simulink model "PN_generator_Tx"  (R2020a)
settings: Solver=FixedStepAuto  StartTime=0.0  StopTime=60  RelTol=1e-3  EnableMultiTasking=on
undefined symbols (not defined in the file): Fs, ip, usb
libraries: commfilt2 x6, commdigbbndpm3 x3, plutoradiolib x2, commseqgen3 x1, commutil2 x1
settings Model: DataTypeOverride=Off  Creator=juanj  LastModifiedBy=juanj
settings SolverCC: PositivePriorityOrder=on
settings OptimizationCC: BlockReduction=off  ConditionallyExecuteInputs=off  EnhancedBackFolding=on  PassReuseOutputArgsAs=Individual arguments  ZeroExternalMemoryAtStartup=off  ZeroInternalMemoryAtStartup=off  MaxStackSize=64  OptimizeBlockOrder=speed  DifferentSizesBufferReuse=on  OptimizationCustomize=off  EfficientTunableParamExpr=on
settings DebuggingCC: SignalRangeChecking=warning  AlgebraicLoopMsg=error  SingleTaskRateTransMsg=error  ParameterTunabilityLossMsg=error  SFUnexpectedBacktrackingDiag=warning  SFNoUnconditionalDefaultTransitionDiag=warning  UnderSpecifiedDimensionMsg=warning
settings HardwareCC: ProdBitPerPointer=32  ProdBitPerSizeT=32  ProdBitPerPtrDiffT=32  ProdLargestAtomicInteger=Long  ProdLargestAtomicFloat=Double  ProdWordSize=32  ProdLongLongMode=on  ProdHWDeviceType=ARM Compatible->ARM Cortex  TargetBitPerPointer=64  TargetBitPerSizeT=64  TargetBitPerPtrDiffT=64  TargetLongLongMode=on  TargetIntDivRoundTo=Zero  TargetEndianess=LittleEndian  TargetWordSize=64  TargetHWDeviceType=Custom Processor->MATLAB Host Computer  ProdEqTarget=off
settings SFSimCC: MATLABDynamicMemAlloc=off
settings RTWCC: SystemTargetFile=ert.tlc  HardwareBoard=ZedBoard  TemplateMakefile=ert_default_tmf  GenerateReport=on  Toolchain=Linaro AArch32 Linux v6.3.1  BuildConfiguration=Debug  LaunchReport=on
settings CodeAppCC: ForceParamTrailComments=on  IgnoreCustomStorageClasses=off  OperatorAnnotations=on  SimulinkDataObjDesc=on  SFDataObjDesc=on  InsertBlockDesc=on  EnableCustomComments=on

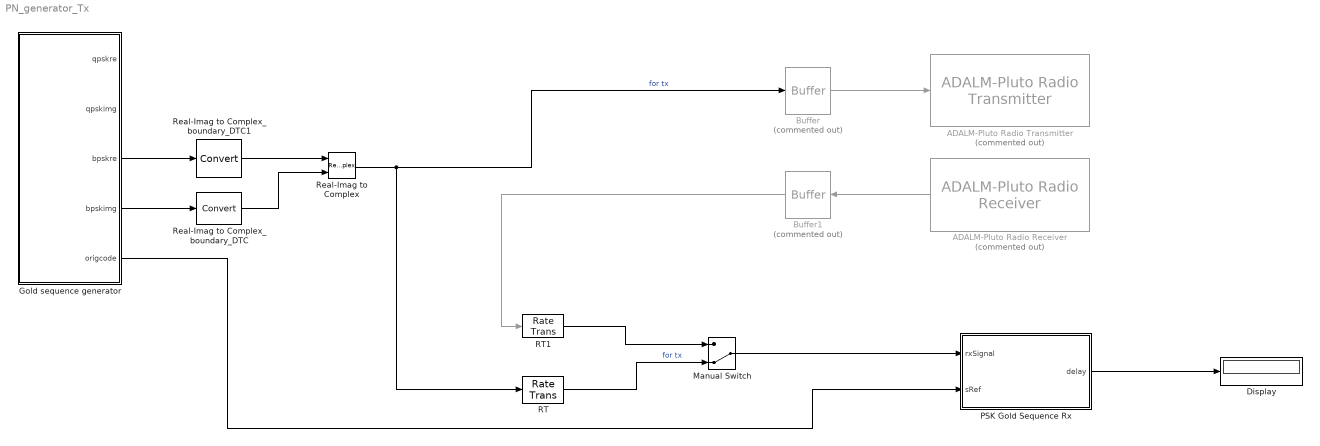
== system PN_generator_Tx ==
  ADALM-Pluto Radio Receiver : plutoradiolib/ADALM-Pluto Radio Receiver  Commented=on  RadioID=usb:0  uri=ip:10.0.0.200  CenterFrequencySource=Dialog  CenterFrequency=900e6  GainSource=AGC Slow Attack  GainSourceBlock=AGC Slow Attack  Gain=10  ChannelMapping=1  BasebandSampleRate=0.5e6  OutputDataType=double  SamplesPerFrame=11216  OverflowOutputPort=off  EnableBurstMode=off  NumFramesInBurst=1  ShowAdvancedProperties=off  UseCustomFilter=off  filtPathRates=[737280000 11520000 3840000 1920000 960000 240000]  filtCoefficients=[-192 82 85 -215 228 -102 -110 290 -318 145 160 -426 471 -215 -238 633 -697 318 349 -923 1009 -457 -498 1309 -1423 640 693 -1812 1959 -876 -945 2458 -2647 1180 1268 -3290 3534 -1572 -1688 4375 -4698 2091 2247 -5836 6284 -2807 -3031 7918 -8588 3870 4225 -11182 12324 -5662 -6330 17255 -19735 9507 11312 -33568 43355 -25227 -42139 305542 305542 -42139 -25227 43355 -33568 11312 9507 -19735 17255 -6330 -5662 12324 -11182 4225 3870 -8588 7918 -3031 -2807 6284 -5836 2247 2091 -4698 4375 -1688 -1572 3534 -3290 1268 1180 -2647 2458 -945 -876 1959 -1812 693 640 -1423 1309 -498 -457 1009 -923 349 318 -697 633 -238 -215 471 -426 160 145 -318 290 -110 -102 228 -215 85 82 -192]  filtCoefficientSize=128  filtDecimInterpFactor=4  filtGain=-12  filtRFBandwidth=18000000  filterConfigStruct=struct()  EnableQuadratureCorrection=on  EnableRFDCCorrection=on  EnableBasebandDCCorrection=on  FrequencyCorrection=0  OverrideSampleTime=off  SampleTime=0.02  DataTimeout=Inf  ENSMPinControlMode=None  BISTLoopbackMode=Disabled  BISTToneInject=Disabled  BISTSignalGen=PRBS  BISTToneFreq=Fs/32  BISTToneLevel=0
      settings: SourceProductBaseCode=PLUTO
  ADALM-Pluto Radio Transmitter : plutoradiolib/ADALM-Pluto Radio Transmitter  Commented=on  RadioID=usb:0  uri=ip:10.0.0.200  CenterFrequencySource=Dialog  CenterFrequency=900e6  GainSource=Dialog  Gain=0  ChannelMapping=1  BasebandSampleRate=0.5e6  UnderflowOutputPort=off  ShowAdvancedProperties=off  UseCustomFilter=off  filtPathRates=[737280000 11520000 3840000 1920000 960000 240000]  filtCoefficients=[-192 82 85 -215 228 -102 -110 290 -318 145 160 -426 471 -215 -238 633 -697 318 349 -923 1009 -457 -498 1309 -1423 640 693 -1812 1959 -876 -945 2458 -2647 1180 1268 -3290 3534 -1572 -1688 4375 -4698 2091 2247 -5836 6284 -2807 -3031 7918 -8588 3870 4225 -11182 12324 -5662 -6330 17255 -19735 9507 11312 -33568 43355 -25227 -42139 305542 305542 -42139 -25227 43355 -33568 11312 9507 -19735 17255 -6330 -5662 12324 -11182 4225 3870 -8588 7918 -3031 -2807 6284 -5836 2247 2091 -4698 4375 -1688 -1572 3534 -3290 1268 1180 -2647 2458 -945 -876 1959 -1812 693 640 -1423 1309 -498 -457 1009 -923 349 318 -697 633 -238 -215 471 -426 160 145 -318 290 -110 -102 228 -215 85 82 -192]  filtCoefficientSize=128  filtDecimInterpFactor=4  filtGain=-12  filtRFBandwidth=18000000  filterConfigStruct=struct()  DataSourceSelect=Input Port  DDSTone1Freq=5e3  DDSTone2Freq=10e3  DDSTone1Scale=0.5  DDSTone2Scale=0.25  DataTimeout=Inf  FrequencyCorrection=0  ENSMPinControlMode=None  BISTLoopbackMode=Disabled  BISTToneInject=Disabled  BISTSignalGen=PRBS  BISTToneFreq=Fs/32  BISTToneLevel=0
      settings: SourceProductBaseCode=PLUTO
  Buffer : Buffer  Commented=on  N=11216  OutputFrames=off
  Buffer1 : Buffer  Commented=on  N=1  OutputFrames=off
  Display : Display
  Gold sequence generator : Subsystem  TreatAsAtomicUnit=on
  Manual Switch : ManualSwitch  CurrentSetting=0
  PSK Gold Sequence Rx : Subsystem
  RT : RateTransition
  RT1 : RateTransition
  Real-Imag to Complex : RealImagToComplex
  Real-Imag to Complex_boundary_DTC : DataTypeConversion  SaturateOnIntegerOverflow=on  RndMeth=Zero
  Real-Imag to Complex_boundary_DTC1 : DataTypeConversion  SaturateOnIntegerOverflow=on  RndMeth=Zero
  wires:
  Real-Imag to Complex/1 -> RT/1, Buffer/1  "for tx"
  Buffer/1 -> ADALM-Pluto Radio Transmitter/1
  Gold sequence generator/4(bpskimg) -> Real-Imag to Complex_boundary_DTC/1
  Real-Imag to Complex_boundary_DTC/1 -> Real-Imag to Complex/2
  Gold sequence generator/3(bpskre) -> Real-Imag to Complex_boundary_DTC1/1
  Real-Imag to Complex_boundary_DTC1/1 -> Real-Imag to Complex/1
  Gold sequence generator/5(origcode) -> PSK Gold Sequence Rx/2(sRef)
  RT/1 -> Manual Switch/2  "for tx"
  ADALM-Pluto Radio Receiver/1 -> Buffer1/1
  Buffer1/1 -> RT1/1
  RT1/1 -> Manual Switch/1
  PSK Gold Sequence Rx/1(delay) -> Display/1
  Manual Switch/1 -> PSK Gold Sequence Rx/1(rxSignal)

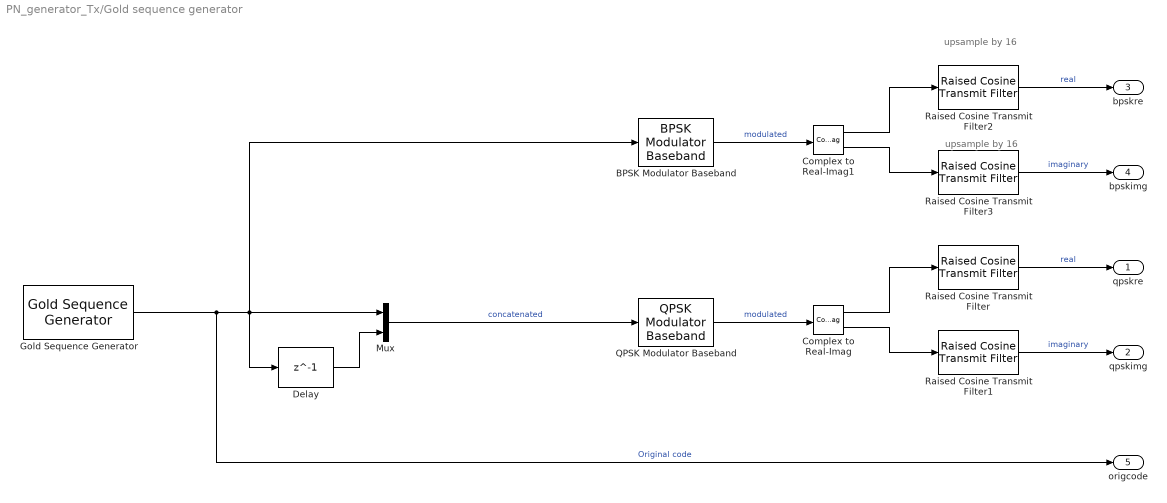
== system PN_generator_Tx/Gold sequence generator ==
  note: upsample by 16
  note: upsample by 16
  BPSK Modulator Baseband : commdigbbndpm3/BPSK Modulator Baseband  Ph=0  outDtype=Fixed-point  outWordLen=16  outUDDataType=sfix(16)  outFracLenMode=Best precision  outFracLen=15  outDataTypeStr=fixdt(1,16)  outLastDataTypeStr=fixdt(1,16)
  Complex to Real-Imag : ComplexToRealImag
  Complex to Real-Imag1 : ComplexToRealImag
  Delay : Delay  DelayLength=1  InitialCondition=0  UseCircularBuffer=on
  Gold Sequence Generator : commseqgen3/Gold Sequence Generator  genPoly1='z^6 + z + 1'  iniState1=[0 1 0 1 0 1]  genPoly2='z^6 + z^5 + z^2 + z + 1'  iniState2=[0 0 0 0 0 1]  index=0  shift=0  outVarSiz=off  maxOutSizeMode=Dialog parameter  maxOutSize=[10 1]  Ts=1/100  sampPerFrame=1  reset=off  outDataType=boolean
      settings: SourceProductBaseCode=CM
  Mux : Mux  Inputs=2
  QPSK Modulator Baseband : commdigbbndpm3/QPSK Modulator Baseband  InType=Bit  Enc=Gray  Ph=pi/4  outDtype=Fixed-point  outWordLen=16  outUDDataType=sfix(16)  outFracLenMode=Best precision  outFracLen=15  outDataTypeStr=fixdt(1,16)  outLastDataTypeStr=fixdt(1,16)
  Raised Cosine Transmit Filter : commfilt2/Raised Cosine Transmit Filter  filtType=Square root  R=0.7  filtSpan=12  N=2  filterGain=1  RateOptions=Allow multirate processing  framing=Mute  checkCoeff=off  variableName=rcTxFilt  checkGain=Normalized  sampMode=Mute  saveAsFlag=0  currentFiltSpan=12  D=(12)/2  launchFVT=on  roundingMode=Floor  overflowMode=off  coeffDataTypeStr=Inherit: Same word length as input  coeffMin=[]  coeffMax=[]  coeffLastDataTypeStr=Inherit: Same word length as input  outputMin=[]  outputMax=[]
  Raised Cosine Transmit Filter1 : commfilt2/Raised Cosine Transmit Filter  filtType=Square root  R=0.7  filtSpan=12  N=2  filterGain=1  RateOptions=Allow multirate processing  framing=Mute  checkCoeff=off  variableName=rcTxFilt1  checkGain=Normalized  sampMode=Mute  saveAsFlag=0  currentFiltSpan=12  D=(12)/2  launchFVT=on  roundingMode=Floor  overflowMode=off  coeffDataTypeStr=Inherit: Same word length as input  coeffMin=[]  coeffMax=[]  coeffLastDataTypeStr=Inherit: Same word length as input  outputMin=[]  outputMax=[]
  Raised Cosine Transmit Filter2 : commfilt2/Raised Cosine Transmit Filter  filtType=Square root  R=0.5  filtSpan=10  N=16  filterGain=1  InputProcessing=Columns as channels (frame based)  RateOptions=Allow multirate processing  framing=Mute  checkCoeff=off  variableName=rcTxFilt2  checkGain=Normalized  sampMode=Mute  saveAsFlag=0  currentFiltSpan=10  D=(10)/2  launchFVT=on  roundingMode=Floor  overflowMode=off  coeffDataTypeStr=Inherit: Same word length as input  coeffMin=[]  coeffMax=[]  coeffLastDataTypeStr=Inherit: Same word length as input  outputMin=[]  outputMax=[]
  Raised Cosine Transmit Filter3 : commfilt2/Raised Cosine Transmit Filter  filtType=Square root  R=0.5  filtSpan=10  N=16  filterGain=1  InputProcessing=Columns as channels (frame based)  RateOptions=Allow multirate processing  framing=Mute  checkCoeff=off  variableName=rcTxFilt3  checkGain=Normalized  sampMode=Mute  saveAsFlag=0  currentFiltSpan=10  D=(10)/2  launchFVT=on  roundingMode=Floor  overflowMode=off  coeffDataTypeStr=Inherit: Same word length as input  coeffMin=[]  coeffMax=[]  coeffLastDataTypeStr=Inherit: Same word length as input  outputMin=[]  outputMax=[]
  qpskre : Outport
  qpskimg : Outport  Port=2  VectorParamsAs1DForOutWhenUnconnected=off
  bpskre : Outport  Port=3
  bpskimg : Outport  Port=4  VectorParamsAs1DForOutWhenUnconnected=off
  origcode : Outport  Port=5
  wires:
  QPSK Modulator Baseband/1 -> Complex to Real-Imag/1  "modulated"
  Raised Cosine Transmit Filter/1 -> qpskre/1  "real"
  Raised Cosine Transmit Filter1/1 -> qpskimg/1  "imaginary"
  Complex to Real-Imag/1 -> Raised Cosine Transmit Filter/1
  Complex to Real-Imag/2 -> Raised Cosine Transmit Filter1/1
  Gold Sequence Generator/1 -> origcode/1, Delay/1, BPSK Modulator Baseband/1, Mux/1  "Original code"
  Mux/1 -> QPSK Modulator Baseband/1  "concatenated"
  Delay/1 -> Mux/2
  Complex to Real-Imag1/1 -> Raised Cosine Transmit Filter2/1
  Raised Cosine Transmit Filter3/1 -> bpskimg/1  "imaginary"
  Raised Cosine Transmit Filter2/1 -> bpskre/1  "real"
  Complex to Real-Imag1/2 -> Raised Cosine Transmit Filter3/1
  BPSK Modulator Baseband/1 -> Complex to Real-Imag1/1  "modulated"

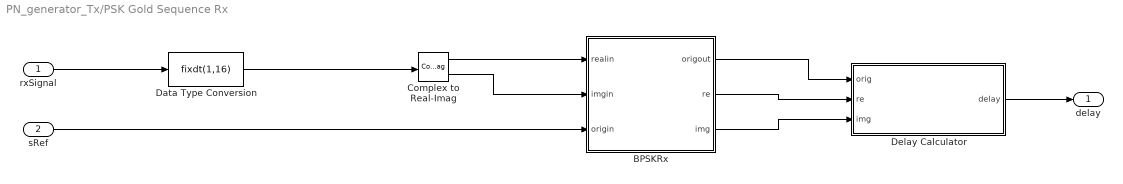
== system PN_generator_Tx/PSK Gold Sequence Rx ==
  rxSignal : Inport
  sRef : Inport  Port=2
  BPSKRx : Subsystem  TreatAsAtomicUnit=on
  Complex to Real-Imag : ComplexToRealImag
  Data Type Conversion : DataTypeConversion  OutMax=[1]  OutDataTypeStr=fixdt(1,16)
  Delay Calculator : Subsystem
  delay : Outport
  wires:
  rxSignal/1 -> Data Type Conversion/1
  sRef/1 -> BPSKRx/3(origin)
  Data Type Conversion/1 -> Complex to Real-Imag/1
  Complex to Real-Imag/2 -> BPSKRx/2(imgin)
  Complex to Real-Imag/1 -> BPSKRx/1(realin)
  BPSKRx/1(origout) -> Delay Calculator/1(orig)
  Delay Calculator/1(delay) -> delay/1
  BPSKRx/2(re) -> Delay Calculator/2(re)
  BPSKRx/3(img) -> Delay Calculator/3(img)

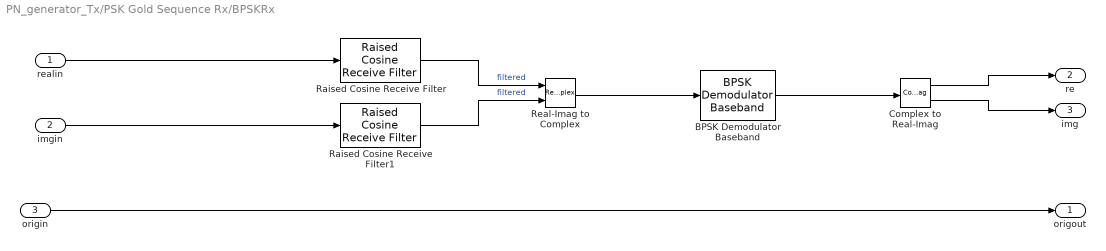
== system PN_generator_Tx/PSK Gold Sequence Rx/BPSKRx ==
  realin : Inport
  imgin : Inport  Port=2
  origin : Inport  Port=3
  BPSK Demodulator Baseband : commdigbbndpm3/BPSK Demodulator Baseband  DecType=Hard decision  VarSource=Dialog  Variance=1  Ph=0  outDtype=Inherit via internal rule  derotateFactorWordLen=16  derotateFactorDataTypeStr=Inherit: Same word length as input  derotateFactorLastDataTypeStr=Inherit: Same word length as input
  Complex to Real-Imag : ComplexToRealImag
  Raised Cosine Receive Filter : commfilt2/Raised Cosine Receive Filter  filtType=Square root  R=0.5  filtSpan=10  N=16  downFactor=16  downOffset=0  filterGain=1  RateOptions=Allow multirate processing  framing=Mute  checkCoeff=off  variableName=rcRxFilt  currentFiltSpan=10  D=5  inputOffset=0  sampMode=Mute  saveAsFlag=0  rateMode=Downsampling  checkGain=Normalized  launchFVT=on  roundingMode=Floor  overflowMode=off  coeffDataTypeStr=Inherit: Same word length as input  coeffMin=[]  coeffMax=[]  coeffLastDataTypeStr=Inherit: Same word length as input  accumDataTypeStr=Inherit: Same as product output  accumLastDataTypeStr=Inherit: Same as product output  outputDataTypeStr=Inherit: Same as accumulator  outputMin=[]  outputMax=[]  outputLastDataTypeStr=Inherit: Same as accumulator
  Raised Cosine Receive Filter1 : commfilt2/Raised Cosine Receive Filter  filtType=Square root  R=0.5  filtSpan=10  N=16  downFactor=16  downOffset=0  filterGain=1  RateOptions=Allow multirate processing  framing=Mute  checkCoeff=off  variableName=rcRxFilt1  currentFiltSpan=10  D=5  inputOffset=0  sampMode=Mute  saveAsFlag=0  rateMode=Downsampling  checkGain=Normalized  launchFVT=on  roundingMode=Floor  overflowMode=off  coeffDataTypeStr=Inherit: Same word length as input  coeffMin=[]  coeffMax=[]  coeffLastDataTypeStr=Inherit: Same word length as input  accumDataTypeStr=Inherit: Same as product output  accumLastDataTypeStr=Inherit: Same as product output  outputDataTypeStr=Inherit: Same as accumulator  outputMin=[]  outputMax=[]  outputLastDataTypeStr=Inherit: Same as accumulator
  Real-Imag to Complex : RealImagToComplex
  origout : Outport
  re : Outport  Port=2
  img : Outport  Port=3
  wires:
  origin/1 -> origout/1
  realin/1 -> Raised Cosine Receive Filter/1
  BPSK Demodulator Baseband/1 -> Complex to Real-Imag/1
  Complex to Real-Imag/1 -> re/1
  Complex to Real-Imag/2 -> img/1
  Real-Imag to Complex/1 -> BPSK Demodulator Baseband/1
  Raised Cosine Receive Filter/1 -> Real-Imag to Complex/1  "filtered"
  Raised Cosine Receive Filter1/1 -> Real-Imag to Complex/2  "filtered"
  imgin/1 -> Raised Cosine Receive Filter1/1

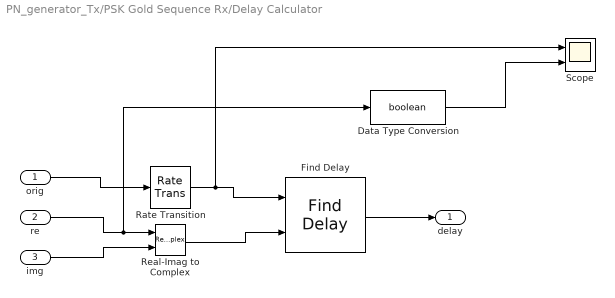
== system PN_generator_Tx/PSK Gold Sequence Rx/Delay Calculator ==
  orig : Inport
  re : Inport  Port=2
  img : Inport  Port=3
  Data Type Conversion : DataTypeConversion  OutDataTypeStr=boolean
  Find Delay : commutil2/Find Delay  corrLength=200  chgSigOP=off  stopUpdate=off  numConstDelay=3
      settings: SourceProductBaseCode=CM
  Rate Transition : RateTransition
  Real-Imag to Complex : RealImagToComplex
  Scope : Scope  NumInputPorts=2
  delay : Outport
  wires:
  Rate Transition/1 -> Scope/1, Find Delay/1
  re/1 -> Data Type Conversion/1, Real-Imag to Complex/1
  Real-Imag to Complex/1 -> Find Delay/2
  Find Delay/1 -> delay/1
  orig/1 -> Rate Transition/1
  img/1 -> Real-Imag to Complex/2
  Data Type Conversion/1 -> Scope/2
